simulink model "winz"  (Simulink 7.9)
settings: Solver=ode3  StartTime=0.0  StopTime=10.0  FixedStep=0.08  RelTol=1e-3
libraries: simulink x2
settings Model: Creator=Daniel  LastModifiedBy=Daniel

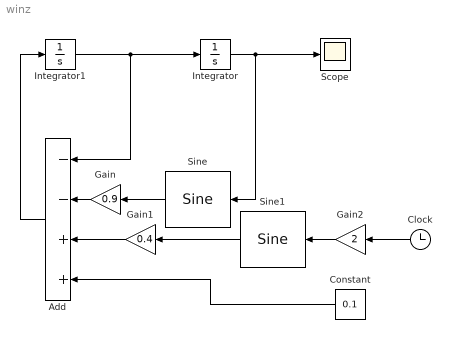
== system winz ==
  Add : Sum  Inputs=--++
  Clock : Clock
  Constant : Constant  Value=0.1
  Gain : Gain  Gain=0.9
  Gain1 : Gain  Gain=0.4
  Gain2 : Gain  Gain=2
  Integrator : Integrator
  Integrator1 : Integrator  InitialCondition=2
  Scope : Scope
  Sine : simulink/Lookup Tables/Sine  Formula=sin(2*pi*u)  NumDataPoints=(2^5)+1  OutputWordLength=16
  Sine1 : simulink/Lookup Tables/Sine  Formula=sin(2*pi*u)  NumDataPoints=(2^5)+1  OutputWordLength=16
  wires:
  Add/1 -> Integrator1/1
  Integrator1/1 -> Integrator/1, Add/1
  Gain/1 -> Add/2
  Integrator/1 -> Sine/1, Scope/1
  Sine/1 -> Gain/1
  Gain1/1 -> Add/3
  Sine1/1 -> Gain1/1
  Gain2/1 -> Sine1/1
  Constant/1 -> Add/4
  Clock/1 -> Gain2/1
